simulink model "a1"  (R2020a)
settings: Solver=VariableStepAuto  StartTime=0.0  StopTime=10.0  RelTol=1e-3
libraries: simulink x1
settings Model: Creator=bill2  LastModifiedBy=bill2
settings DataIOCC: Refine=10

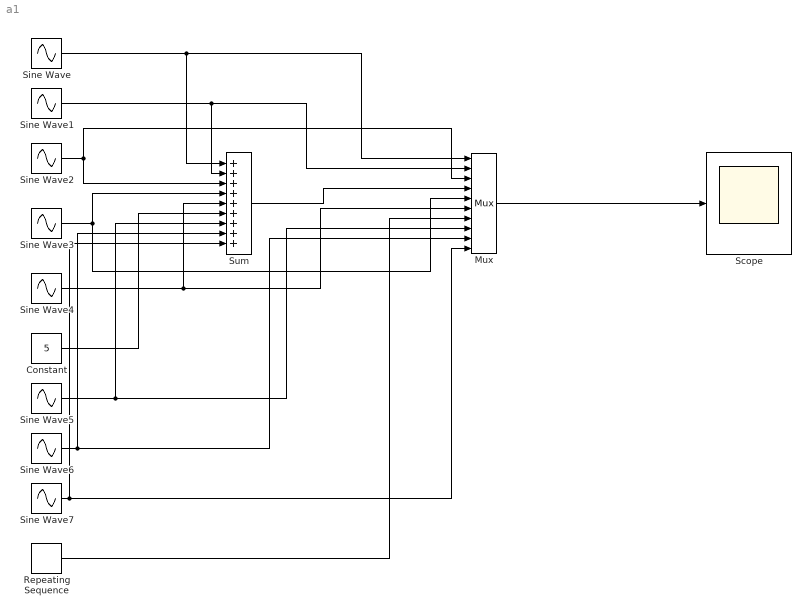
== system a1 ==
  Constant : Constant  Value=5
  Mux : Mux  Inputs=10
  Repeating Sequence : simulink/Sources/Repeating Sequence  rep_seq_t=[0 2]  rep_seq_y=[0 10]
  Scope : Scope
  Sine Wave : Sin  Amplitude=-10/pi  Frequency=pi  SampleTime=0
  Sine Wave1 : Sin  Amplitude=-10/(2*pi)  Frequency=2*pi  SampleTime=0
  Sine Wave2 : Sin  Amplitude=-10/(3*pi)  Frequency=3*pi  SampleTime=0
  Sine Wave3 : Sin  Amplitude=-10/(4*pi)  Frequency=4*pi  SampleTime=0
  Sine Wave4 : Sin  Amplitude=-10/(5*pi)  Frequency=5*pi  SampleTime=0
  Sine Wave5 : Sin  Amplitude=-10/(6*pi)  Frequency=6*pi  SampleTime=0
  Sine Wave6 : Sin  Amplitude=-10/(7*pi)  Frequency=7*pi  SampleTime=0
  Sine Wave7 : Sin  Amplitude=-10/(8*pi)  Frequency=8*pi  SampleTime=0
  Sum : Sum  Inputs=9
  wires:
  Sine Wave2/1 -> Mux/3, Sum/3
  Sine Wave3/1 -> Mux/5, Sum/4
  Sine Wave4/1 -> Mux/6, Sum/5
  Constant/1 -> Sum/6
  Sum/1 -> Mux/4
  Sine Wave/1 -> Mux/1, Sum/1
  Sine Wave1/1 -> Sum/2, Mux/2
  Repeating Sequence/1 -> Mux/7
  Mux/1 -> Scope/1
  Sine Wave5/1 -> Mux/8, Sum/7
  Sine Wave6/1 -> Mux/9, Sum/8
  Sine Wave7/1 -> Mux/10, Sum/9
